simulink model "Drone_UAVScenario"  (R2025a)
settings: Solver=VariableStepAuto  StartTime=0.0  StopTime=10  RelTol=1e-3
values from neighbouring files (symbols this model uses):
  envData = Simulink.Bus.createMATLABStruct('MultirotorGuidanceEnvironmentBus')    [setup_drone.m]
  waypoints = [0 0 -2; 10 0 -2; 10 10 -2; 0 10 -2; 0 0 -2]    [setup_drone.m]
libraries: uavalgslib x2, uavutilslib x1
settings Model: PacingRate=1000  Creator=siddx  LastModifiedBy=siddx

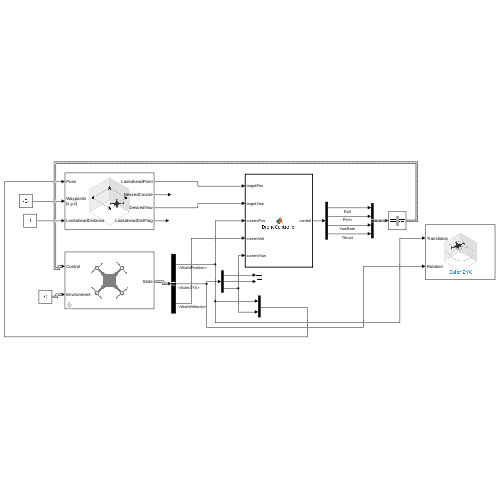
[thumbnail: Simulink's stored preview of the top-level diagram]
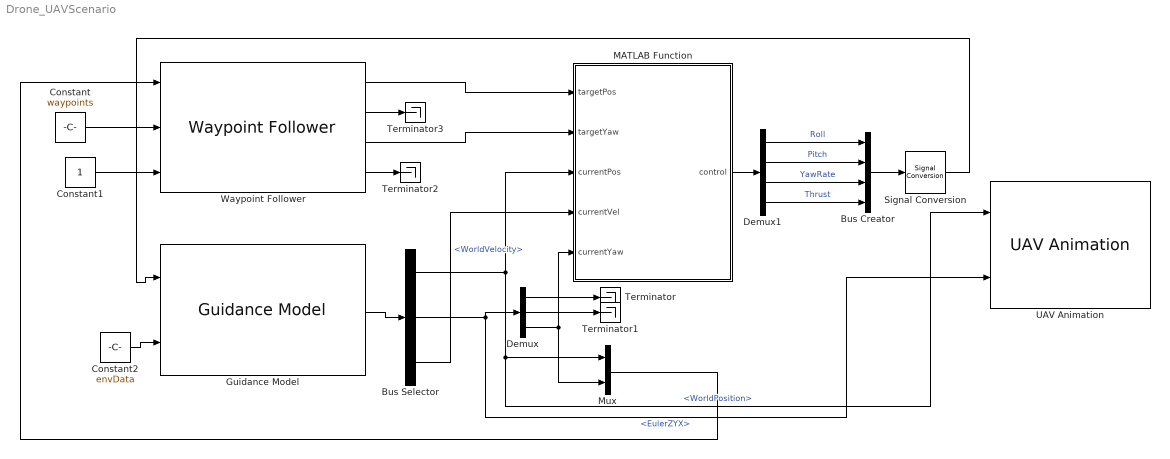
== system Drone_UAVScenario ==
  Bus Creator : BusCreator  Inputs=4  OutDataTypeStr=Bus: MultirotorGuidanceControlBus  NonVirtualBus=on
  Bus Selector : BusSelector  OutputSignals=WorldPosition,EulerZYX,WorldVelocity
  Constant : Constant  Value=waypoints
  Constant1 : Constant
  Constant2 : Constant  Value=envData  OutDataTypeStr=Bus: MultirotorGuidanceEnvironmentBus
  Demux : Demux  Outputs=3
  Demux1 : Demux
  Guidance Model : uavalgslib/Guidance Model  ModelType=MultirotorGuidance  NumInstances=1  SpecifiedDataType=double  SimulateUsing=Interpreted execution  InitialWorldPositionMultirotor=[0; 0; 0]  InitialWorldVelocityMultirotor=[0; 0; 0]  InitialEulerZYXMultirotor=[0; 0; 0]  InitialBodyAngularRateRPYMultirotor=[0; 0; 0]  InitialThrustMultirotor=0  InitialNorthFixedWing=0  InitialEastFixedWing=0  InitialHeightFixedWing=0  InitialAirSpeedFixedWing=0  InitialHeadingAngleFixedWing=0  InitialFlightPathAngleFixedWing=0  InitialRollAngleFixedWing=0  InitialRollAngleRateFixedWing=0  PDRollMultirotor=[3402.97,116.67]  PDPitchMultirotor=[3402.97, 116.67]  PYawRateMultirotor=1950  PThrustMultirotor=3900  MassMultirotor=2.83  PHeightFixedWing=3.9  PHeadingAngleFixedWing=3.9  PFlightPathAngleFixedWing=39  PDRollFixedWing=[3402.97, 116.67]  PAirSpeedFixedWing=1  FlightPathAngleLimitsFixedWing=[-pi/2, pi/2]  StateBusName='MultirotorGuidanceStateBus'  ControlBusName='MultirotorGuidanceControlBus'  EnvironmentBusName='MultirotorGuidanceEnvironmentBus'  DataType=double
      link override ControlSignalSpecification: OutDataTypeStr=Bus: MultirotorGuidanceControlBus
      link override EnvironmentSignalSpecification: OutDataTypeStr=Bus: MultirotorGuidanceEnvironmentBus
  MATLAB Function : MATLAB Function  TreatAsAtomicUnit=on
  Mux : Mux  Inputs=2
  Signal Conversion : SignalConversion  ConversionOutput=Nonvirtual bus  OutDataTypeStr=Bus: MultirotorGuidanceControlBus  OverrideOpt=off
  Terminator{,1..3} (4 alike) : Terminator
  UAV Animation : uavutilslib/UAV Animation  NumUAV=1  DynamicUAVConfig=off  UAVType=Multirotor  UAVSize=1  UAVColor=[1 0 0]  UAVTrajectoryAlpha=1  InertialZDirection=Down  RotationFormat=Euler ZYX  DrawMarkers=off  SampleTime=-1
  Waypoint Follower : uavalgslib/Waypoint Follower  UAVType=multirotor  StartFrom=first  TransitionRadiusSource=internal  TransitionRadius=1  MinLookaheadDistance=1  HoverAtLastWaypoint=on  YawInput=off  ShowCrossTrackErrorOutput=off  ShowStatusOutput=off  SimulateUsing=Interpreted execution
  wires:
  Constant/1 -> Waypoint Follower/2
  Waypoint Follower/1 -> MATLAB Function/1(targetPos)
  Waypoint Follower/3 -> MATLAB Function/2(targetYaw)
  Guidance Model/1 -> Bus Selector/1
  Bus Selector/1 -> UAV Animation/1, Mux/1, MATLAB Function/3(currentPos)  "<WorldPosition>"
  Bus Selector/3 -> MATLAB Function/4(currentVel)  "<WorldVelocity>"
  Bus Selector/2 -> UAV Animation/2, Demux/1  "<EulerZYX>"
  Demux/3 -> Mux/2, MATLAB Function/5(currentYaw)
  Demux/1 -> Terminator/1
  Demux/2 -> Terminator1/1
  Mux/1 -> Waypoint Follower/1
  Constant1/1 -> Waypoint Follower/3
  Constant2/1 -> Guidance Model/2
  Waypoint Follower/4 -> Terminator2/1
  MATLAB Function/1(control) -> Demux1/1
  Demux1/1 -> Bus Creator/1  "Roll"
  Demux1/2 -> Bus Creator/2  "Pitch"
  Demux1/3 -> Bus Creator/3  "YawRate"
  Demux1/4 -> Bus Creator/4  "Thrust"
  Bus Creator/1 -> Signal Conversion/1
  Signal Conversion/1 -> Guidance Model/1
  Waypoint Follower/2 -> Terminator3/1

== matlab function Drone_UAVScenario/MATLAB Function ==
  data: targetPos input; control output; targetYaw input; currentPos input; currentVel input; currentYaw input
function control = DroneController(targetPos, targetYaw, currentPos, currentVel, currentYaw)
    % DRONE CONFIGURATION
    mass = 2.83;     % kg
    g = 9.81;        % Gravity
    
    % PID GAINS (Reduced for stability)
    Kp_xy = 1.5;     % Position P
    Kd_xy = 1.2;     % Velocity D (Damping)
    Kp_z  = 4.0;     % Altitude P (Stronger)
    Kd_z  = 2.5;     % Altitude D
    Kp_yaw = 1.5;    % Yaw P (Positive standard)

    % 1. POSITION ERRORS
    posErr = targetPos - currentPos;
    
    % 2. DESIRED VELOCITY
    % Limit the max tilt/speed to prevent flipping
    velDes = posErr * Kp_xy;
    maxSpeed = 5;
    if norm(velDes) > maxSpeed
        velDes = (velDes / norm(velDes)) * maxSpeed;
    end
    
    % 3. DESIRED ACCELERATION
    accDes = (velDes - currentVel) * Kd_xy;
    
    % Altitude Control (PD)
    % accDes(3) will be negative if we want to go UP (NED frame)
    accDes(3) = (posErr(3) * Kp_z) - (currentVel(3) * Kd_z);

    % 4. CONVERT TO BODY FRAME (Roll/Pitch)
    psi = currentYaw;
    rotation = [cos(psi) sin(psi); -sin(psi) cos(psi)];
    bodyAcc = rotation * [accDes(1); accDes(2)];
    
    % Pitch controls X-body accel, Roll controls Y-body accel
    cmdPitch = -bodyAcc(1) / g; 
    cmdRoll  =  bodyAcc(2) / g;
    
    % Clamp Angles (Safety: Don't tilt more than 30 degrees)
    maxTilt = 0.5; % radians (~30 deg)
    cmdPitch = max(min(cmdPitch, maxTilt), -maxTilt);
    cmdRoll = max(min(cmdRoll, maxTilt), -maxTilt);
    
    % 5. CALCULATE THRUST (FIXED FORMULA)
    % NED Frame: F_net = m*a = m*g - Thrust
    % Therefore: Thrust = m * (g - a_z)
    cmdThrust = mass * (g - accDes(3));
    
    % 6. YAW CONTROL
    yawErr = targetYaw - currentYaw;
    % Normalize angle to -pi to pi
    while yawErr > pi, yawErr = yawErr - 2*pi; end
    while yawErr < -pi, yawErr = yawErr + 2*pi; end
    cmdYawRate = yawErr * Kp_yaw;

    % OUTPUT
    control = [cmdRoll, cmdPitch, cmdYawRate, cmdThrust];
end
